simulink model "cpu2_mc_algorithm"  (R2020a)
settings: Solver=FixedStepDiscrete  StartTime=0.0  StopTime=inf  RelTol=1e-3  EnableMultiTasking=on
values from neighbouring files (symbols this model uses):
  CurAOffset = 2238.0    [cpu2_mc_algorithm.sldd]
  CurBOffset = 2250.0    [cpu2_mc_algorithm.sldd]
  CurCOffset = 2260.0    [cpu2_mc_algorithm.sldd]
  CurScale = 0.012    [cpu2_mc_algorithm.sldd]
  Ls = 0.00025    [cpu2_mc_algorithm.sldd]
  RATIO = 100.0    [cpu2_mc_algorithm.sldd]
  Rs = 0.15    [cpu2_mc_algorithm.sldd]
undefined symbols (not defined in the file or in its folder): C28x, CPU1, CPU2, DiscIntNeverNeededParam, Down, GPTRIP1SEL, GPTRIP2SEL, sawtooth, TZ1, TZ2, Up
libraries: c2802xlib x9, c2837xDlib x6, simulink x4, c2000lib x1
(part 2 of 2)

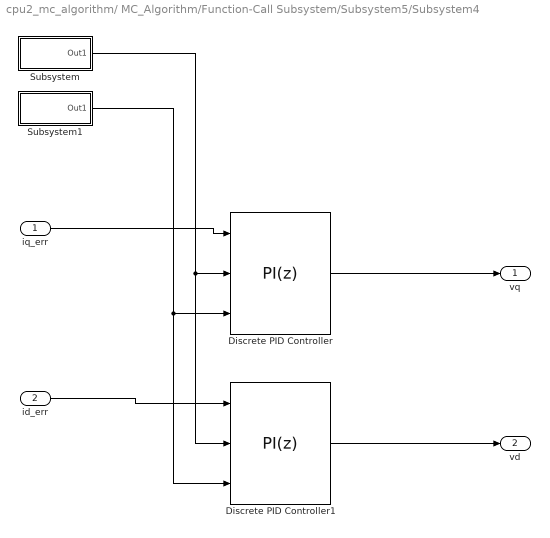
== system cpu2_mc_algorithm/ MC_Algorithm/Function-Call Subsystem/Subsystem5/Subsystem4 ==
  iq_err : Inport
  id_err : Inport  Port=2
  Discrete PID Controller : simulink/Continuous/PID Controller  Controller=PI  Form=Parallel  TimeDomain=Discrete-time  UseExternalTs=off  SampleTime=-1  IntegratorMethod=Forward Euler  FilterMethod=Forward Euler  ControllerParametersSource=external  P=Ls*1000  I=Rs*1000  D=0  UseFilter=on  N=100  TunerSelectOption=Transfer Function Based (PID Tuner App)  ZeroCross=off  InitialConditionSource=internal  InitialConditionForIntegrator=0  InitialConditionForFilter=0  DifferentiatorICPrevScaledInput=0  ExternalReset=none  TrackingMode=off  Kt=1  LimitOutput=on  UpperSaturationLimit=9  LowerSaturationLimit=-9  LinearizeAsGain=off  AntiWindupMode=clamping  Kb=Ls/Rs  PGainOutDataTypeStr=single  PProdOutDataTypeStr=single  POutMin=[]  POutMax=[]  IGainOutDataTypeStr=single  IProdOutDataTypeStr=single  IOutMin=[]  IOutMax=[]  DOutMin=[]  DOutMax=[]  NOutMin=[]  NOutMax=[]  SumOutDataTypeStr=single  SumOutMin=[]  SumOutMax=[]  SaturationOutDataTypeStr=single  SaturationOutMin=-9  SaturationOutMax=9  PParamMin=[]  PParamMax=[]  IParamMin=[]  IParamMax=[]  DParamMin=[]  DParamMax=[]  NParamMin=[]  NParamMax=[]  KbParamMin=[]  KbParamMax=[]  KtParamMin=[]  KtParamMax=[]  KbOutMin=[]  KbOutMax=[]  KtOutMin=[]  KtOutMax=[]  IntegratorOutMin=[]  IntegratorOutMax=[]  FilterOutMin=[]  FilterOutMax=[]  SumI1OutMin=[]  SumI1OutMax=[]  SumI2OutMin=[]  SumI2OutMax=[]  SumI3OutMin=[]  SumI3OutMax=[]  SumI4OutMin=[]  SumI4OutMax=[]  SumDOutMin=[]  SumDOutMax=[]  DifferentiatorOutMin=[]  DifferentiatorOutMax=[]  FilterDiffOutCoefMin=[]  FilterDiffOutCoefMax=[]  ReciprocalOutMin=[]  ReciprocalOutMax=[]  SumDenOutMin=[]  SumDenOutMax=[]  SumNumOutMin=[]  SumNumOutMax=[]  DivideOutMin=[]  DivideOutMax=[]  UdiffTsProdOutMin=[]  UdiffTsProdOutMax=[]  NTsProdOutMin=[]  NTsProdOutMax=[]  UintegralTsProdOutMin=[]  UintegralTsProdOutMax=[]  UngainTsProdOutMin=[]  UngainTsProdOutMax=[]  IntegratorContinuousStateAttributes=''  IntegratorStateMustResolveToSignalObject=off  IntegratorRTWStateStorageClass=Auto  FilterContinuousStateAttributes=''  FilterStateMustResolveToSignalObject=off  FilterRTWStateStorageClass=Auto  ParallelPVariant=ExternalParameters  IdealPVariant=Disabled  IVariant=ExternalParameters  DVariant=Disabled  IntegratorVariant=Discrete  SatVariant=Enabled  AWVariant=DiscClampingParallel  PCopyVariant=Disabled  TRVariant=Disabled  FdbkBlocksVariant=Forward  IdealPFdbkVariant=Disabled  SatFdbkVariant=Disabled  DerivativeFilterVariant=Disabled  NVariant=Disabled  NCopyVariant=Disabled_SignalSpec  FilterICVariant=Disabled  IntegratorICVariant=InternalICs  ExternalResetVariant=Disabled  TRSumVariant=Passthrough  SumFdbkVariant=Disabled  SumVariant=Sum_PI  TsampFilterVariant=InternalTs  TsampNgainVariant=Passthrough  TsampIntegralVariant=Passthrough
  Discrete PID Controller1 : simulink/Continuous/PID Controller  Controller=PI  Form=Parallel  TimeDomain=Discrete-time  UseExternalTs=off  SampleTime=-1  IntegratorMethod=Forward Euler  FilterMethod=Forward Euler  ControllerParametersSource=external  P=Ls*1000  I=Rs*1000  D=0  UseFilter=on  N=100  TunerSelectOption=Transfer Function Based (PID Tuner App)  ZeroCross=off  InitialConditionSource=internal  InitialConditionForIntegrator=0  InitialConditionForFilter=0  DifferentiatorICPrevScaledInput=0  ExternalReset=none  TrackingMode=off  Kt=1  LimitOutput=on  UpperSaturationLimit=9  LowerSaturationLimit=-9  LinearizeAsGain=off  AntiWindupMode=clamping  Kb=Ls/Rs  PGainOutDataTypeStr=single  PProdOutDataTypeStr=single  POutMin=[]  POutMax=[]  IGainOutDataTypeStr=single  IProdOutDataTypeStr=single  IOutMin=[]  IOutMax=[]  DOutMin=[]  DOutMax=[]  NOutMin=[]  NOutMax=[]  SumOutDataTypeStr=single  SumOutMin=[]  SumOutMax=[]  SaturationOutDataTypeStr=single  SaturationOutMin=-9  SaturationOutMax=9  PParamMin=[]  PParamMax=[]  IParamMin=[]  IParamMax=[]  DParamMin=[]  DParamMax=[]  NParamMin=[]  NParamMax=[]  KbParamMin=[]  KbParamMax=[]  KtParamMin=[]  KtParamMax=[]  KbOutMin=[]  KbOutMax=[]  KtOutMin=[]  KtOutMax=[]  IntegratorOutMin=[]  IntegratorOutMax=[]  FilterOutMin=[]  FilterOutMax=[]  SumI1OutMin=[]  SumI1OutMax=[]  SumI2OutMin=[]  SumI2OutMax=[]  SumI3OutMin=[]  SumI3OutMax=[]  SumI4OutMin=[]  SumI4OutMax=[]  SumDOutMin=[]  SumDOutMax=[]  DifferentiatorOutMin=[]  DifferentiatorOutMax=[]  FilterDiffOutCoefMin=[]  FilterDiffOutCoefMax=[]  ReciprocalOutMin=[]  ReciprocalOutMax=[]  SumDenOutMin=[]  SumDenOutMax=[]  SumNumOutMin=[]  SumNumOutMax=[]  DivideOutMin=[]  DivideOutMax=[]  UdiffTsProdOutMin=[]  UdiffTsProdOutMax=[]  NTsProdOutMin=[]  NTsProdOutMax=[]  UintegralTsProdOutMin=[]  UintegralTsProdOutMax=[]  UngainTsProdOutMin=[]  UngainTsProdOutMax=[]  IntegratorContinuousStateAttributes=''  IntegratorStateMustResolveToSignalObject=off  IntegratorRTWStateStorageClass=Auto  FilterContinuousStateAttributes=''  FilterStateMustResolveToSignalObject=off  FilterRTWStateStorageClass=Auto  ParallelPVariant=ExternalParameters  IdealPVariant=Disabled  IVariant=ExternalParameters  DVariant=Disabled  IntegratorVariant=Discrete  SatVariant=Enabled  AWVariant=DiscClampingParallel  PCopyVariant=Disabled  TRVariant=Disabled  FdbkBlocksVariant=Forward  IdealPFdbkVariant=Disabled  SatFdbkVariant=Disabled  DerivativeFilterVariant=Disabled  NVariant=Disabled  NCopyVariant=Disabled_SignalSpec  FilterICVariant=Disabled  IntegratorICVariant=InternalICs  ExternalResetVariant=Disabled  TRSumVariant=Passthrough  SumFdbkVariant=Disabled  SumVariant=Sum_PI  TsampFilterVariant=InternalTs  TsampNgainVariant=Passthrough  TsampIntegralVariant=Passthrough
  Subsystem : Subsystem
      mask Display: disp("Ls * RATIO")
  Subsystem1 : Subsystem
      mask Display: disp("Rs * RATIO")
  vq : Outport  VectorParamsAs1DForOutWhenUnconnected=off
  vd : Outport  Port=2  VectorParamsAs1DForOutWhenUnconnected=off
  wires:
  id_err/1 -> Discrete PID Controller1/1
  iq_err/1 -> Discrete PID Controller/1
  Subsystem/1(Out1) -> Discrete PID Controller/2, Discrete PID Controller1/2
  Subsystem1/1(Out1) -> Discrete PID Controller1/3, Discrete PID Controller/3
  Discrete PID Controller/1 -> vq/1
  Discrete PID Controller1/1 -> vd/1

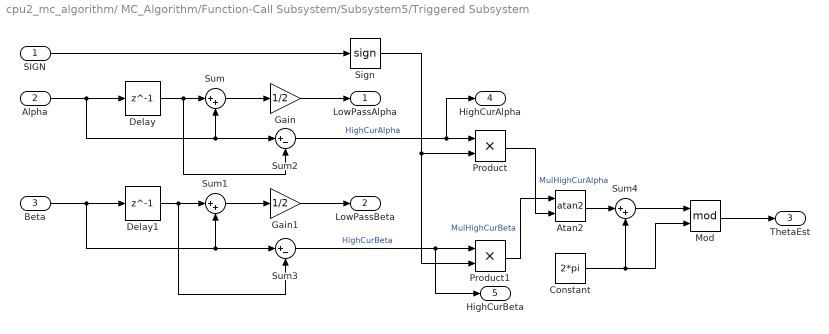
== system cpu2_mc_algorithm/ MC_Algorithm/Function-Call Subsystem/Subsystem5/Triggered Subsystem ==
  SIGN : Inport
  Alpha : Inport  Port=2
  Beta : Inport  Port=3
  Atan2 : Trigonometry  Operator=atan2
  Constant : Constant  Value=2*pi  OutDataTypeStr=single  SampleTime=-1
  Delay : Delay  DelayLength=1
  Delay1 : Delay  DelayLength=1
  Gain : Gain  Gain=1/2
  Gain1 : Gain  Gain=1/2
  Mod : Math  Operator=mod  SaturateOnIntegerOverflow=on
  Product : Product
  Product1 : Product
  Sign : Signum
  Sum : Sum  Inputs=|++
  Sum1 : Sum  Inputs=|++
  Sum2 : Sum  Inputs=|+-
  Sum3 : Sum  Inputs=|+-
  Sum4 : Sum  Inputs=|++
  LowPassAlpha : Outport  OutDataTypeStr=single
  LowPassBeta : Outport  Port=2  OutDataTypeStr=single
  ThetaEst : Outport  Port=3  OutDataTypeStr=single  InitialOutput=[0]
  HighCurAlpha : Outport  Port=4  OutDataTypeStr=single
  HighCurBeta : Outport  Port=5  OutDataTypeStr=single
  wires:
  Alpha/1 -> Delay/1, Sum/2, Sum2/1
  Delay/1 -> Sum2/2, Sum/1
  Sum/1 -> Gain/1
  Gain/1 -> LowPassAlpha/1
  Sum1/1 -> Gain1/1
  Delay1/1 -> Sum3/2, Sum1/1
  Beta/1 -> Delay1/1, Sum1/2, Sum3/1
  Gain1/1 -> LowPassBeta/1
  SIGN/1 -> Sign/1
  Sum2/1 -> HighCurAlpha/1, Product/1  "HighCurAlpha"
  Sign/1 -> Product/2, Product1/2
  Sum3/1 -> HighCurBeta/1, Product1/1  "HighCurBeta"
  Product/1 -> Atan2/2  "MulHighCurAlpha"
  Product1/1 -> Atan2/1  "MulHighCurBeta"
  Atan2/1 -> Sum4/1
  Constant/1 -> Sum4/2, Mod/2
  Mod/1 -> ThetaEst/1
  Sum4/1 -> Mod/1

== system cpu2_mc_algorithm/ MC_Algorithm/Function-Call Subsystem/Subsystem5/Subsystem1/Subsystem ==
  In1 : Inport
  If : If  IfExpression=u1 > 0.78  ElseIfExpressions=u1 < -0.78
  If Action Subsystem : Subsystem  TreatAsAtomicUnit=on
  If Action Subsystem1 : Subsystem  TreatAsAtomicUnit=on
  If Action Subsystem2 : Subsystem  TreatAsAtomicUnit=on
  Merge : Merge  Inputs=3
  Output : Outport
  wires:
  In1/1 -> If Action Subsystem2/1(In1), If/1
  If/1 -> If Action Subsystem/Action
  If/2 -> If Action Subsystem1/Action
  If/3 -> If Action Subsystem2/Action
  If Action Subsystem/1(Out1) -> Merge/1
  If Action Subsystem1/1(Out1) -> Merge/2
  If Action Subsystem2/1(Out1) -> Merge/3
  Merge/1 -> Output/1

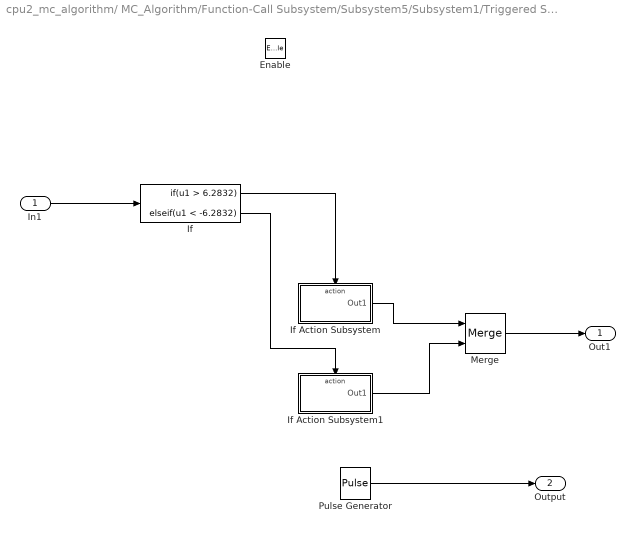
== system cpu2_mc_algorithm/ MC_Algorithm/Function-Call Subsystem/Subsystem5/Subsystem1/Triggered Subsystem ==
  In1 : Inport  OutDataTypeStr=single
  Enable : EnablePort
  If : If  IfExpression=u1 > 6.2832  ElseIfExpressions=u1 < -6.2832  ShowElse=off
  If Action Subsystem : Subsystem  TreatAsAtomicUnit=on
  If Action Subsystem1 : Subsystem  TreatAsAtomicUnit=on
  Merge : Merge
  Pulse Generator : DiscretePulseGenerator  SampleTime=-1
  Out1 : Outport
  Output : Outport  Port=2
  wires:
  In1/1 -> If/1
  If/1 -> If Action Subsystem/Action
  If Action Subsystem/1(Out1) -> Merge/1
  If/2 -> If Action Subsystem1/Action
  If Action Subsystem1/1(Out1) -> Merge/2
  Merge/1 -> Out1/1
  Pulse Generator/1 -> Output/1

== system cpu2_mc_algorithm/ MC_Algorithm/Function-Call Subsystem/Subsystem5/Subsystem4/Subsystem ==
  Constant : Constant  Value=RATIO  OutDataTypeStr=single  SampleTime=-1
  Constant1 : Constant  Value=Ls  SampleTime=-1
  Multiply : Product
  Out1 : Outport  VectorParamsAs1DForOutWhenUnconnected=off
  wires:
  Constant1/1 -> Multiply/1
  Constant/1 -> Multiply/2
  Multiply/1 -> Out1/1

== system cpu2_mc_algorithm/ MC_Algorithm/Function-Call Subsystem/Subsystem5/Subsystem4/Subsystem1 ==
  Constant : Constant  Value=RATIO  SampleTime=-1
  Constant1 : Constant  Value=Rs  OutDataTypeStr=single  SampleTime=-1
  Multiply : Product
  Out1 : Outport  VectorParamsAs1DForOutWhenUnconnected=off
  wires:
  Multiply/1 -> Out1/1
  Constant/1 -> Multiply/2
  Constant1/1 -> Multiply/1

== system cpu2_mc_algorithm/ MC_Algorithm/Function-Call Subsystem/Subsystem5/Subsystem1/Subsystem/If Action Subsystem ==
  Action Port : ActionPort  ActionPortLabel=if(u1 > 0.78)
  Constant : Constant  Value=0  OutDataTypeStr=single
  Out1 : Outport
  wires:
  Constant/1 -> Out1/1

== system cpu2_mc_algorithm/ MC_Algorithm/Function-Call Subsystem/Subsystem5/Subsystem1/Subsystem/If Action Subsystem1 ==
  Action Port : ActionPort  ActionPortLabel=elseif(u1 < -0.78)
  Constant : Constant  Value=0  OutDataTypeStr=single
  Out1 : Outport
  wires:
  Constant/1 -> Out1/1

== system cpu2_mc_algorithm/ MC_Algorithm/Function-Call Subsystem/Subsystem5/Subsystem1/Subsystem/If Action Subsystem2 ==
  In1 : Inport
  Action Port : ActionPort  ActionPortLabel=else
  Out1 : Outport
  wires:
  In1/1 -> Out1/1

== system cpu2_mc_algorithm/ MC_Algorithm/Function-Call Subsystem/Subsystem5/Subsystem1/Triggered Subsystem/If Action Subsystem ==
  Action Port : ActionPort  ActionPortLabel=if(u1 > 6.2832)
  Constant : Constant  Value=pi  OutDataTypeStr=single
  Out1 : Outport
  wires:
  Constant/1 -> Out1/1

== system cpu2_mc_algorithm/ MC_Algorithm/Function-Call Subsystem/Subsystem5/Subsystem1/Triggered Subsystem/If Action Subsystem1 ==
  Action Port : ActionPort  ActionPortLabel=elseif(u1 < -6.2832)
  Constant : Constant  Value=-pi  OutDataTypeStr=single
  Out1 : Outport
  wires:
  Constant/1 -> Out1/1

== stateflow chart cpu2_mc_algorithm/ MC_Algorithm/Function-Call Subsystem/Subsystem5/Chart ==
  state Identify
    state IdentifyDefault
      en:
      id = 0;
      iq = 0;
    state End
      en:
      id = 0;
      du:
      OutTheta = ThetaEst;
      iq = iqRef;
    state IdentifyPos
      en:
      id = 5;
      iq = 0;
      OutTheta = 0.7854; % 45
    state IdentifyPolarity2
      en:
      id = 0;
      iq = 0;
      du:
      OutTheta = ThetaEst;
    state IdentifyPolarity1
      en:
      id = 0;
      iq = 0;
      du:
      OutTheta = ThetaEst;
    state IdentifyPolarity3
      en:
      id = 0;
      iq = 0;
      du:
      OutTheta = ThetaEst;
    (default) -> IdentifyDefault
    IdentifyDefault -> IdentifyPos
    IdentifyPolarity1 -> IdentifyPolarity2 : after(20,msec)
    IdentifyPolarity2 -> IdentifyPolarity3 : after(20,msec)
    IdentifyPos -> IdentifyPolarity1 : after(3,sec)
    IdentifyPolarity3 -> End : after(20,msec)
  (default) -> Identify
  data: iq output single =0; id output single =0; ThetaEst input single; OutTheta output single; iqRef input single
